simulink library "ADRC"  (Simulink 7.6)
settings: Solver=ode45  StartTime=0.0  StopTime=10.0  RelTol=1e-3
values from neighbouring files (symbols this model uses):
  a = x2+y/h    [ADRC_1.m]    (also in ADRC_2.m; ADRC_2fal.m; ADRC_2fal00.m; ADRC_3.m)
  d = r*h    [ADRC_1.m]    (also in ADRC_2.m; ADRC_2fal.m; ADRC_2fal00.m; ADRC_3.m)
  r = [1 1 linspace(0.8,0,9)]'    [Birthday_gift.m]
undefined symbols (not defined in the file or in its folder): A, b, B, Bet, Bet0, Beta1, Beta2, c, D, h, h0, h1, h2, r0, r1, r2
settings Model: Creator=Administrator  LastModifiedBy=Administrator

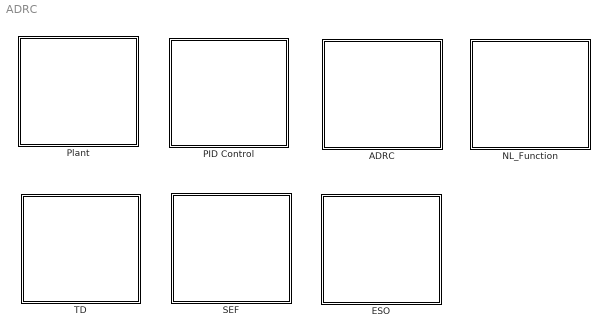
== system ADRC ==
  ADRC : Subsystem
  ESO : Subsystem
  NL_Function : Subsystem
  PID Control : Subsystem
  Plant : Subsystem
  SEF : Subsystem
  TD : Subsystem

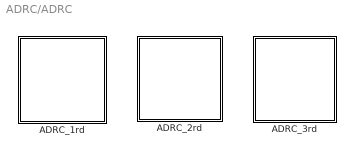
== system ADRC/ADRC ==
  ADRC_1rd : Subsystem
  ADRC_2rd : Subsystem
  ADRC_3rd : Subsystem

== system ADRC/ESO ==
  ESO_2rd : Subsystem
  ESO_3rd : Subsystem
  ESO_4rd : Subsystem

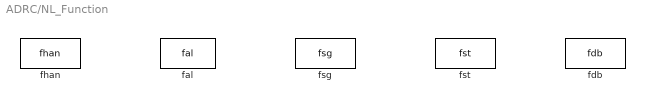
== system ADRC/NL_Function ==
  fal : S-Function  FunctionName=fal  Parameters=a,d  EnableBusSupport=off
  fdb : S-Function  FunctionName=fdb  Parameters=a,b  EnableBusSupport=off
  fhan : S-Function  FunctionName=fhan  Parameters=r,h  EnableBusSupport=off
  fsg : S-Function  FunctionName=fsg  Parameters=a,b  EnableBusSupport=off
  fst : S-Function  FunctionName=fst  Parameters=a,b  EnableBusSupport=off

== system ADRC/PID Control ==
  LinearPID : Subsystem
  NLPID : Subsystem

== system ADRC/Plant ==
  One Order Plant : Subsystem
  Three Order Plant : Subsystem
  Two Order Plant : Subsystem

== system ADRC/SEF ==
  LSEF : Subsystem
  NLSEF : Subsystem

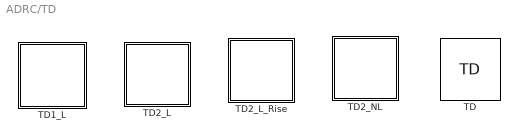
== system ADRC/TD ==
  TD : S-Function  FunctionName=TD  Parameters=r0,h  EnableBusSupport=off  mask{r0=20, h=0.01}
      mask prompts: r0 "r0="; h "h="
  TD1_L : Subsystem
  TD2_L : Subsystem
  TD2_L_Rise : Subsystem
  TD2_NL : Subsystem

== system ADRC/ADRC/ADRC_1rd ==
  ADRC_1rd : Subsystem  mask{r0=0.01, h=0.01, B01=100, B02=2000, r=10}
      mask prompts: r0 "r0="; h "h="; B01 "B01="; B02 "B02="; r "r="

== system ADRC/ADRC/ADRC_2rd ==
  ADRC_2_fal : Subsystem  AncestorBlock=ADRC/ADRC/ADRC_2rd/ADRC_2_order  mask{r=0.01, h=0.01, B01=100, B02=300, B03=1000, D=0.01, b=1, k1=10, k2=5, Ds=0.01}
      mask prompts: B01 "B01="; B02 "B02="; B03 "B03="; D "D="; k1 "k1="; k2 "k2="; Ds "Ds="
  ADRC_2_fhan : Subsystem  mask{h=0.01, TD=[2,0.01], ESO=[100,300,1000,0.01], NLSEF=[0.3,5,0.03], b0=1}
      mask prompts: h "h="; TD "TD[r0,h]="; ESO "ESO[B01,B02,B03,D]="; NLSEF "NLSEF[c,r1,h1]="; b0 "b0="

== system ADRC/ADRC/ADRC_3rd ==
  ADRC_3RD_fal : Subsystem  AncestorBlock=ADRC/ADRC/ADRC_3rd/ADRC_2_fhan/Subsystem  mask{h=0.01, TD=[0.5,0.01], ESO=[100,300,3000,20000], NLSEF=[2,5,4,0.01], b0=1}
      mask prompts: h "h="; TD "TD[r0,h1]="; ESO "ESO[B01,B02,B03,B04,h2]="; NLSEF "NLSEF[K1,K2,K3]"; b0 "b0="
  ADRC_3RD_linear : Subsystem  AncestorBlock=ADRC/ADRC/ADRC_3rd/ADRC_3RD_fal  mask{r=0.5, h=0.01, ESO=[100,3000,30000,200000], NLSEF=[2,5,4], b0=1}
      mask prompts: r "r="; h "h="; ESO "ESO[B01,B02,B03,B04]="; NLSEF "NLSEF[K1,K2,K3]"; b0 "b0="

== system ADRC/ESO/ESO_2rd ==
  ESO_2rd : S-Function  FunctionName=ESO_2rd  Parameters=d,bet,b  EnableBusSupport=off  mask{d=0, b=0, bet=0}
      mask prompts: d "d="; b "b="; bet "bet="

== system ADRC/ESO/ESO_3rd ==
  ESO_2rd1 : S-Function  FunctionName=ESO_3rd  Parameters=d,bet,b  EnableBusSupport=off  mask{d=0, bet=0}
      mask prompts: d "d="; bet "bet="

== system ADRC/ESO/ESO_4rd ==
  ESO_2L : Subsystem  mask{bet=[100 65 82], b=1}
      mask prompts: bet "bet=[]"; b "b="

== system ADRC/PID Control/LinearPID ==
  S-Function1 : S-Function  FunctionName=Linear_PD  Parameters=Beta1,Beta2,h  EnableBusSupport=off
  S-Function4 : S-Function  FunctionName=Linear_PID_TD1_SO  Parameters=r0,h,B,Bet,D  EnableBusSupport=off
  S-Function5 : S-Function  FunctionName=Linear_PID_2LinearTD  Parameters=r0,r1,h,Bet  EnableBusSupport=off

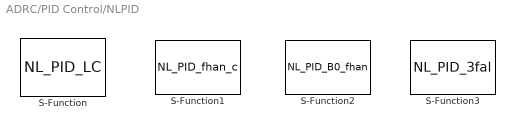
== system ADRC/PID Control/NLPID ==
  S-Function : S-Function  FunctionName=NL_PID_LC  Parameters=r0,h0,r1,h1,h,Bet  EnableBusSupport=off
  S-Function1 : S-Function  FunctionName=NL_PID_fhan_c  Parameters=r0,h0,r1,h1,h,c,r2,h2  EnableBusSupport=off
  S-Function2 : S-Function  FunctionName=NL_PID_B0_fhan  Parameters=r0,h0,r1,h1,h,Bet0,r2,h2  EnableBusSupport=off
  S-Function3 : S-Function  FunctionName=NL_PID_3fal  Parameters=r0,h0,r1,h1,h,Bet,A,D  EnableBusSupport=off

== system ADRC/Plant/One Order Plant ==
  One Order Plant : S-Function  EnableBusSupport=off

== system ADRC/Plant/Three Order Plant ==
  Three Order Plant : S-Function  FunctionName=Plant3  EnableBusSupport=off

== system ADRC/Plant/Two Order Plant ==
  Two  Order  Plant : S-Function  FunctionName=Plant1_x1x2wt  EnableBusSupport=off
  Two Order  Plant : S-Function  FunctionName=Plant1_x1x2  EnableBusSupport=off
  Two Order Plant : S-Function  FunctionName=Plant1_fhan  EnableBusSupport=off

== system ADRC/SEF/LSEF ==
  NLSFS1 : S-Function  FunctionName=NLSFS1  EnableBusSupport=off
  NLSFS2 : S-Function  FunctionName=NLSFS1  EnableBusSupport=off

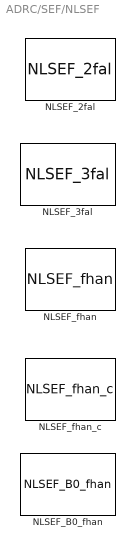
== system ADRC/SEF/NLSEF ==
  NLSEF_2fal : S-Function  FunctionName=NLSEF_2fal  Parameters=Beta1,A1,Beta2,A2,Delta  EnableBusSupport=off  mask{Beta1=80, Beta2=50, A1=0.25, A2=0.5, Delta=0.02}
      mask prompts: Beta1 "Beta1="; Beta2 "Beta2="; A1 "A1="; A2 "A2="; Delta "Delta="
  NLSEF_3fal : S-Function  FunctionName=NLSEF_3fal  Parameters=B,A,Delta  EnableBusSupport=off  mask{B=[10,5,100], A=[0.25,0.75,1.5], Delta=0.02}
      mask prompts: B "B=[ ; ; ]"; A "A=[ ; ; ]"
  NLSEF_B0_fhan : S-Function  FunctionName=NLSEF_B0_fhan  Parameters=Beta0,r1,h1  EnableBusSupport=off  mask{Beta0=500, r1=20, h1=0.08}
      mask prompts: Beta0 "Beta0="; r1 "r1="; h1 "h1="
  NLSEF_fhan : S-Function  FunctionName=NLSEF_fhan  Parameters=r,h1  EnableBusSupport=off  mask{r=30, h1=0.08}
      mask prompts: r "r="; h1 "h1="
  NLSEF_fhan_c : S-Function  FunctionName=NLSEF_fhan_c  Parameters=c,r2,h2  EnableBusSupport=off  mask{c=1, r2=30, h2=0.08}
      mask prompts: c "c="; r2 "r2="; h2 "h2="

== system ADRC/TD/TD1_L ==
  TD1_L : S-Function  FunctionName=TD1_L  Parameters=RisingTime,SampleTime  EnableBusSupport=off  mask{RisingTime=5, SampleTime=0.01}
      mask prompts: RisingTime "RisingTime="; SampleTime "SampleTime="

== system ADRC/TD/TD2_L ==
  TD2_L : S-Function  FunctionName=TD2_L  Parameters=r,h  EnableBusSupport=off  mask{r=5, h=0.01}
      mask prompts: r "r="; h "h="

== system ADRC/TD/TD2_L_Rise ==
  TD2_L_Rise : S-Function  FunctionName=TD2_L_Rise  Parameters=RisingTime,SampleTime  EnableBusSupport=off  mask{RisingTime=5, SampleTime=0.004}
      mask prompts: RisingTime "RisingTime="

== system ADRC/TD/TD2_NL ==
  TD2_NL : S-Function  FunctionName=TD2_NL  Parameters=r,h,h0  EnableBusSupport=off  mask{r=20, h=0.01, h0=0.01}
      mask prompts: r "r="; h "h="; h0 "h0="

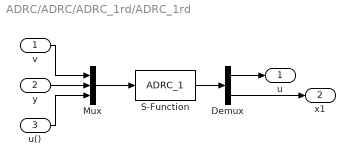
== system ADRC/ADRC/ADRC_1rd/ADRC_1rd ==
  v : Inport
  y : Inport  Port=2
  u() : Inport  Port=3
  Demux : Demux  Outputs=2
  Mux : Mux  Inputs=3
  S-Function : S-Function  FunctionName=ADRC_1  Parameters=r0,h,B01,B02,r  EnableBusSupport=off
  u : Outport
  x1 : Outport  Port=2
  wires:
  v/1 -> Mux/1
  y/1 -> Mux/2
  Mux/1 -> S-Function/1
  u()/1 -> Mux/3
  S-Function/1 -> Demux/1
  Demux/1 -> u/1
  Demux/2 -> x1/1

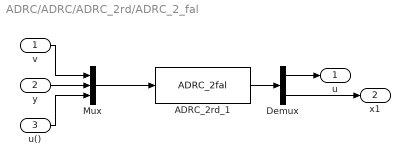
== system ADRC/ADRC/ADRC_2rd/ADRC_2_fal ==
  v : Inport
  y : Inport  Port=2
  u() : Inport  Port=3
  ADRC_2rd_1 : S-Function  FunctionName=ADRC_2fal  Parameters=r,h,B01,B02,B03,D,b,k1,k2,Ds  EnableBusSupport=off
  Demux : Demux  Outputs=2
  Mux : Mux  Inputs=3
  u : Outport
  x1 : Outport  Port=2
  wires:
  u()/1 -> Mux/3
  Mux/1 -> ADRC_2rd_1/1
  y/1 -> Mux/2
  v/1 -> Mux/1
  ADRC_2rd_1/1 -> Demux/1
  Demux/1 -> u/1
  Demux/2 -> x1/1

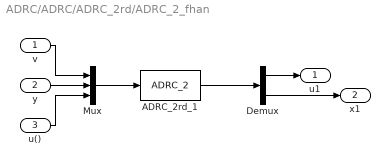
== system ADRC/ADRC/ADRC_2rd/ADRC_2_fhan ==
  v : Inport
  y : Inport  Port=2
  u() : Inport  Port=3
  ADRC_2rd_1 : S-Function  FunctionName=ADRC_2  Parameters=h,TD,ESO,NLSEF,b0  EnableBusSupport=off
  Demux : Demux  Outputs=2
  Mux : Mux  Inputs=3
  u1 : Outport
  x1 : Outport  Port=2
  wires:
  v/1 -> Mux/1
  y/1 -> Mux/2
  Mux/1 -> ADRC_2rd_1/1
  u()/1 -> Mux/3
  ADRC_2rd_1/1 -> Demux/1
  Demux/1 -> u1/1
  Demux/2 -> x1/1

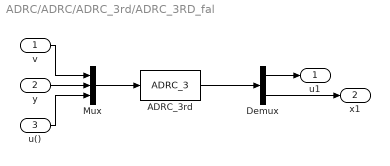
== system ADRC/ADRC/ADRC_3rd/ADRC_3RD_fal ==
  v : Inport
  y : Inport  Port=2
  u() : Inport  Port=3
  ADRC_3rd : S-Function  FunctionName=ADRC_3  Parameters=h,TD,ESO,NLSEF,b0  EnableBusSupport=off
  Demux : Demux  Outputs=2
  Mux : Mux  Inputs=3
  u1 : Outport
  x1 : Outport  Port=2
  wires:
  Demux/2 -> x1/1
  Demux/1 -> u1/1
  ADRC_3rd/1 -> Demux/1
  u()/1 -> Mux/3
  Mux/1 -> ADRC_3rd/1
  y/1 -> Mux/2
  v/1 -> Mux/1

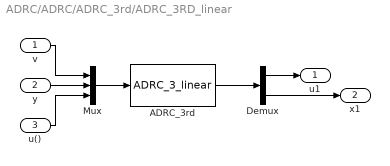
== system ADRC/ADRC/ADRC_3rd/ADRC_3RD_linear ==
  v : Inport
  y : Inport  Port=2
  u() : Inport  Port=3
  ADRC_3rd : S-Function  FunctionName=ADRC_3_linear  Parameters=r,h,ESO,NLSEF,b0  EnableBusSupport=off
  Demux : Demux  Outputs=2
  Mux : Mux  Inputs=3
  u1 : Outport
  x1 : Outport  Port=2
  wires:
  v/1 -> Mux/1
  y/1 -> Mux/2
  Mux/1 -> ADRC_3rd/1
  u()/1 -> Mux/3
  ADRC_3rd/1 -> Demux/1
  Demux/1 -> u1/1
  Demux/2 -> x1/1

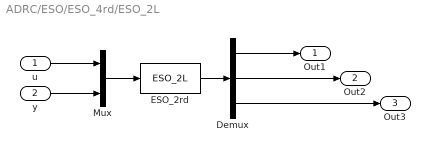
== system ADRC/ESO/ESO_4rd/ESO_2L ==
  u : Inport
  y : Inport  Port=2
  Demux : Demux  Outputs=3
  ESO_2rd : S-Function  FunctionName=ESO_2L  Parameters=bet,b  EnableBusSupport=off
  Mux : Mux  Inputs=2
  Out1 : Outport
  Out2 : Outport  Port=2
  Out3 : Outport  Port=3
  wires:
  y/1 -> Mux/2
  Mux/1 -> ESO_2rd/1
  ESO_2rd/1 -> Demux/1
  Demux/1 -> Out1/1
  Demux/2 -> Out2/1
  Demux/3 -> Out3/1
  u/1 -> Mux/1
